simulink model "InnerOuter_Sim"  (Simulink 6.6)
settings: Solver=ode4  StartTime=0.0  StopTime=125  FixedStep=SampleT  RelTol=1e-3
InitFcn:
  | clc
  | innerOuterInit
undefined symbols (not defined in the file): A1, Apolar, apSampleTime, bankCommandLimit, baseHeight, baseTemp, CD0, chord, CL0, CLa, CLa_dot, Clb, ClDa, CLDe, CLDf, ClDr, clock, Clp, CLq, Clr, Cm0, Cma, CmDe, CmDf, Cmq, Cnb, CnDa, CnDr, Cnp, Cnr, compensatorOn, CYb, CYDr, da_failamp, da_failbias, da_failper, daL_fail, daLimit, daR_fail, deg, deLimit, derivativesConstant, dr_fail, dr_failamp, dr_failbias, dr_failper, drLimit, dtLimit, Earth, elarm, Euler_0, F, gaind, getWP, ISA_g, Ixx, Iyy, Izz, L1OF, L2_base ... (+28)
libraries: simulink x102, SLUGS_Library x23, aerolibconvert2 x15, dsPICdrivers x8, aerolibactuator x5, aerolibtransform2 x2, aerolibwind2 x2, dspmtrx3 x2, aerolibatmos2 x1, aerolibutil x1
(part 3 of 4)

== system InnerOuter_Sim/L1 Output Feedback Controller With  Projection Operator/State Predictor/Compute Coef ==
  a : Inport
  Enable : EnablePort
  -T : Gain  Gain=-apSampleTime  SampleTime=apSampleTime
  1-c : Sum  Inputs=-+  OutDataTypeMode=single  OutScaling=2^-10
  Constant : Constant
  Subsystem11 : Subsystem  AncestorBlock=SLUGS_Library/Subsystem11
  b : Outport
  c : Outport  Port=2
  wires:
  -T/1 -> Subsystem11/1(u)
  Subsystem11/1(exp(u)) -> 1-c/1, c/1  "c"
  Constant/1 -> 1-c/2
  1-c/1 -> b/1
  a/1 -> -T/1

== system InnerOuter_Sim/L1 Output Feedback Controller With  Projection Operator/State Predictor/Detect Change ==
  Data : Inport
  Abs1 : Abs  SampleTime=apSampleTime
  Difference1 : simulink/Discrete/Difference  SystemSampleTime=-1  ICPrevInput=0.0  OutDataType=sfix(16)  OutScaling=2^-10  DoSatur=off
  Saturation1 : Saturate  UpperLimit=1  LowerLimit=0  SampleTime=apSampleTime
  change? : Outport
  wires:
  Difference1/1 -> Abs1/1
  Abs1/1 -> Saturation1/1
  Data/1 -> Difference1/1
  Saturation1/1 -> change?/1

== system InnerOuter_Sim/L1 Output Feedback Controller With  Projection Operator/Trapezoidal Integrator/Protect NaNs ==
  In1 : Inport
  Integer Delay3 : simulink/Discrete/Integer Delay  Orientation=left  vinit=0.0  samptime=T  NumDelays=1
  Relational Operator2 : RelationalOperator  Operator===  LogicOutDataTypeMode=Specify via dialog
  Switch3 : Switch  Criteria=u2 > Threshold  Threshold=0.3  SampleTime=.01
  Out1 : Outport  Orientation=down
  wires:
  Integer Delay3/1 -> Switch3/3
  Switch3/1 -> Out1/1, Integer Delay3/1
  In1/1 -> Relational Operator2/2, Relational Operator2/1, Switch3/1
  Relational Operator2/1 -> Switch3/2

== system InnerOuter_Sim/L1 Output Feedback Controller With  Projection Operator/Trapezoidal Integrator/Protect NaNs1 ==
  In1 : Inport
  Integer Delay3 : simulink/Discrete/Integer Delay  Orientation=left  vinit=0.0  samptime=T  NumDelays=1
  Relational Operator2 : RelationalOperator  Operator===  LogicOutDataTypeMode=Specify via dialog
  Switch3 : Switch  Criteria=u2 > Threshold  Threshold=0.3  SampleTime=.01
  Out1 : Outport  Orientation=down
  wires:
  Relational Operator2/1 -> Switch3/2
  In1/1 -> Switch3/1, Relational Operator2/1, Relational Operator2/2
  Switch3/1 -> Integer Delay3/1, Out1/1
  Integer Delay3/1 -> Switch3/3

== system InnerOuter_Sim/Lateral Channel/Sideslip Compensation/Bank to Psi Dot ==
  phi_c : Inport
  U_m : Inport  Port=2
  Constant1 : Constant  Value=9.80665  OutDataTypeMode=single
  Divide : Product  Inputs=/*  OutDataTypeMode=single  OutScaling=2^-10  SampleTime=apSampleTime
  Divide1 : Product  OutDataTypeMode=single  OutScaling=2^-10  SampleTime=apSampleTime
  Subsystem8 : SLUGS_Library/Subsystem8  SystemSampleTime=-1
  negprotect : Stateflow chart
  psi_dot_c : Outport
  wires:
  negprotect/1(zpVal) -> Divide/1
  Divide/1 -> Divide1/2
  phi_c/1 -> Subsystem8/1
  Subsystem8/1 -> Divide1/1
  Divide1/1 -> psi_dot_c/1
  Constant1/1 -> Divide/2
  U_m/1 -> negprotect/1(val)

== system InnerOuter_Sim/Lateral Channel/Sideslip Compensation/Low Pass ==
  a : Inport
  u : Inport  Port=2
  Compute Coef : Subsystem
  Detect Change : Subsystem
  Divide : Product  OutScaling=2^-10  SampleTime=apSampleTime
  Divide1 : Product  OutScaling=2^-10  SampleTime=apSampleTime
  IC : InitialCondition
  Integer Delay : simulink/Discrete/Integer Delay  vinit=0.0  samptime=apSampleTime  NumDelays=1
  Integer Delay1 : simulink/Discrete/Integer Delay  Orientation=left  vinit=0.0  samptime=apSampleTime  NumDelays=1
  Subtract : Sum  OutScaling=2^-10  SampleTime=apSampleTime
  y : Outport
  wires:
  a/1 -> Compute Coef/1(a), Detect Change/1(Data)
  Compute Coef/1(b) -> Divide/1
  Compute Coef/2(c) -> Divide1/1
  Detect Change/1(change?) -> IC/1
  Integer Delay/1 -> Divide/2
  Divide/1 -> Subtract/1
  Divide1/1 -> Subtract/2
  Subtract/1 -> y/1, Integer Delay1/1
  IC/1 -> Compute Coef/Enable
  u/1 -> Integer Delay/1
  Integer Delay1/1 -> Divide1/2

== system InnerOuter_Sim/Lateral Channel/Sideslip Compensation/psi_dot to Bank ==
  psi_dot_c : Inport
  U_m : Inport  Port=2
  Constant1 : Constant  Value=9.80665  OutDataTypeMode=single
  Divide : Product  Inputs=**/  OutScaling=2^-10  SampleTime=apSampleTime
  Subsystem2 : SLUGS_Library/Subsystem2  SystemSampleTime=-1
  phi_c : Outport
  wires:
  Divide/1 -> Subsystem2/1
  Subsystem2/1 -> phi_c/1
  Constant1/1 -> Divide/3
  U_m/1 -> Divide/2
  psi_dot_c/1 -> Divide/1

== system InnerOuter_Sim/Longitudinal Channel/Airspeed Hold [PID]/Trapezoidal Integrator ==
  x : Inport
  Reset : Inport  Port=2
  Constant : Constant  Value=1/3  OutDataTypeMode=single
  Constant1 : Constant  Value=4/3  OutDataTypeMode=single
  Constant2 : Constant  Value=T/2  OutDataTypeMode=single
  Constant3 : Constant  Value=1/3  OutDataTypeMode=single
  Constant5 : Constant  Orientation=left  Value=0  OutDataTypeMode=single
  Integer Delay : simulink/Discrete/Integer Delay  vinit=0.0  samptime=T  NumDelays=1
  Integer Delay1 : simulink/Discrete/Integer Delay  vinit=0.0  samptime=T  NumDelays=2
  Integer Delay2 : simulink/Discrete/Integer Delay  Orientation=left  vinit=0.0  samptime=T  NumDelays=1
  Product{,1..3} (4 alike) : Product  OutDataTypeMode=single  RndMeth=Zero
  "Protect NaNs " : Subsystem
  Protect NaNs1 : Subsystem
  Subtract : Sum  Inputs=3  OutDataTypeMode=single  OutScaling=2^-10
  Subtract1 : Sum  Inputs=2  OutDataTypeMode=single  OutScaling=2^-10
  Switch1 : Switch  Criteria=u2 > Threshold  Threshold=0.3  SampleTime=.01
  Int(x) : Outport
  wires:
  Switch1/1 -> Protect NaNs1/1(In1)
  Reset/1 -> Switch1/2
  Constant5/1 -> Switch1/1
  Product3/1 -> Subtract1/2
  Integer Delay2/1 -> Subtract1/1
  Subtract1/1 -> Switch1/3
  Subtract/1 -> Product3/2
  Constant2/1 -> Product3/1
  Product2/1 -> Subtract/3
  Product1/1 -> Subtract/2
  Product/1 -> Subtract/1
  x/1 -> "Protect NaNs "/1(In1)
  Constant3/1 -> Product2/2
  Integer Delay1/1 -> Product2/1
  Integer Delay/1 -> Product1/1
  Constant1/1 -> Product1/2
  Constant/1 -> Product/2
  Protect NaNs1/1(Out1) -> Integer Delay2/1, Int(x)/1
  "Protect NaNs "/1(Out1) -> Integer Delay1/1, Integer Delay/1, Product/1

== system InnerOuter_Sim/Navigation/Compute WP Switching Trigger/Compute  Projection ==
  Puav : Inport
  WP0 : Inport  Port=2
  T : Inport  Port=3
  Protect NaNs : Subsystem
  Subsystem3 : Subsystem  AncestorBlock=SLUGS_Library/Subsystem3
  Subtract : Sum  Inputs=+-  OutDataTypeMode=single  OutScaling=2^-10
  Dg : Outport
  wires:
  Protect NaNs/1(Out1) -> Dg/1
  Puav/1 -> Subtract/1
  WP0/1 -> Subtract/2
  Subtract/1 -> Subsystem3/1(x)
  T/1 -> Subsystem3/2(y)
  Subsystem3/1(x dot y) -> Protect NaNs/1(In1)

== system InnerOuter_Sim/Navigation/Leg Run Computation/Compute Lateral Error ==
  N1 : Inport
  WP0 : Inport  Port=2
  Puav : Inport  Port=3
  Add : Sum  Inputs=+-  OutScaling=2^-10
  Subsystem3 : SLUGS_Library/Subsystem3  SystemSampleTime=-1
  Pe_y : Outport
  wires:
  Subsystem3/1 -> Pe_y/1
  Add/1 -> Subsystem3/2
  N1/1 -> Subsystem3/1
  Puav/1 -> Add/2
  WP0/1 -> Add/1

== system InnerOuter_Sim/Navigation/Leg Run Computation/GainSchedule L2 and Get Groundspeed ==
  L2 Base : Inport
  Vxyz : Inport  Port=2
  Divide4 : Product  OutScaling=2^-10
  "Norm 2 (Consider Only XY) " : Subsystem  AncestorBlock=SLUGS_Library/Navigation/Norm
  To Workspace3 : ToWorkspace  VariableName=L2  SampleTime=-1  SaveFormat=Array
  L2 : Outport
  Groundspeed : Outport  Port=2
  wires:
  "Norm 2 (Consider Only XY) "/1(Norm) -> Groundspeed/1, Divide4/2
  Vxyz/1 -> "Norm 2 (Consider Only XY) "/1(Vector)
  L2 Base/1 -> Divide4/1
  Divide4/1 -> L2/1, To Workspace3/1

== system InnerOuter_Sim/Navigation/Leg Run Computation/Pey <= |L2| (Park and Deyst's) ==
  Pey : Inport
  Vxyz : Inport  Port=2
  L2 : Inport  Port=3
  T1 : Inport  Port=4
  Groundspeed : Inport  Port=5
  Puav : Inport  Port=6
  N1 : Inport  Port=7
  Enable : EnablePort
  Add : Sum  Inputs=+-  OutScaling=2^-10
  Compute D : Subsystem
  Compute Eta : Subsystem
  Gravity1 : Constant  Orientation=left  Value=ISA_g  OutDataTypeMode=single
  Zero out Z : Stateflow chart
  as_c to phi_c1 : Subsystem  AncestorBlock=SLUGS_Library/Navigation/as_c to phi_c
  phi_c : Outport
  L2Vec : Outport  Port=2
  as_c : Outport  Port=3
  wires:
  Compute D/1(D) -> Add/1
  Zero out Z/1(P) -> Add/2, Compute D/4(Puav)
  Vxyz/1 -> Compute Eta/1(Vxyz)
  Add/1 -> Compute Eta/2(L2vec), L2Vec/1
  Gravity1/1 -> as_c to phi_c1/2(g)
  Compute Eta/1(a_s_c) -> as_c to phi_c1/1(as_c), as_c/1
  Pey/1 -> Compute D/1(Pe_y)
  L2/1 -> Compute D/2(|L2|), Compute Eta/4(|L2|)
  Puav/1 -> Zero out Z/1(Pin)
  T1/1 -> Compute D/3(T1)
  Groundspeed/1 -> Compute Eta/3(Groundspeed)
  as_c to phi_c1/1(phi_c) -> phi_c/1
  N1/1 -> Compute D/5(N1)

== system InnerOuter_Sim/Navigation/Leg Run Computation/Pey > |L2| (Marius') ==
  Pey : Inport
  Kr : Inport  Port=2
  T1 : Inport  Port=3
  Tot Run : Inport  Port=4
  Puav : Inport  Port=5
  WP0 : Inport  Port=6
  U_m : Inport  Port=7
  Enable : EnablePort
  Add1 : Sum  Inputs=+-  OutScaling=2^-10
  Add2 : Sum  Inputs=-+  OutScaling=2^-10
  Add3 : Sum  Inputs=-+  OutScaling=2^-10
  Constant1 : Constant  Value=0.0025  OutDataTypeMode=single
  Low_passed Time  Derivative : Subsystem  AncestorBlock="SLUGS_Library/Control Blocks/PD Controller  Internal Derivative/Low_passed Time Derivative"
  Low_passed Time  Derivative1 : Subsystem  AncestorBlock="SLUGS_Library/Control Blocks/PD Controller  Internal Derivative/Low_passed Time Derivative"
  Product : Product  Inputs=3  RndMeth=Zero
  Product1 : Product  RndMeth=Zero
  Product2 : Product  RndMeth=Zero
  Subsystem3 : SLUGS_Library/Subsystem3  SystemSampleTime=-1
  Zero out Z : Stateflow chart
  Zero out Z1 : Stateflow chart
  psi_dot to Bank : Subsystem  AncestorBlock=SLUGS_Library/Navigation/psi_dot to Bank
  phi_c : Outport
  wires:
  Puav/1 -> Add1/1
  WP0/1 -> Add1/2
  Add1/1 -> Zero out Z1/1(Pin)
  T1/1 -> Zero out Z/1(Pin)
  Tot Run/1 -> Add2/2
  psi_dot to Bank/1(phi_c) -> phi_c/1
  Add2/1 -> Product/1, Low_passed Time  Derivative/1(f(t))  "xTrack"
  Pey/1 -> Product1/2, Low_passed Time  Derivative1/1(f(t))  "yTreack"
  Low_passed Time  Derivative1/1(f_dot(t)) -> Product/2
  Kr/1 -> Product/3
  Low_passed Time  Derivative/1(f_dot(t)) -> Product1/1
  Product1/1 -> Add3/1
  Product/1 -> Add3/2
  U_m/1 -> psi_dot to Bank/2(U_m)
  Subsystem3/1 -> Add2/1
  Zero out Z/1(P) -> Subsystem3/1  "Pex"
  Zero out Z1/1(P) -> Subsystem3/2
  Product2/1 -> psi_dot to Bank/1(psi_dot_c)
  Add3/1 -> Product2/2
  Constant1/1 -> Product2/1

== system InnerOuter_Sim/Navigation/Leg Run Computation/Record Data ==
  ApMode : Inport
  "L2Vec " : Inport  Port=2
  as_c : Inport  Port=3
  "ApMode " : InportShadow  Port=1  LatchByCopyingInsideSignal=off
  Constant2 : Constant  Value=[0 0 0]  OutDataTypeMode=single
  Switch : Switch  Threshold=0.3
  Switch1 : Switch  Threshold=0.3
  L2Vec : Outport
  "as_c " : Outport  Port=2
  wires:
  Switch/1 -> L2Vec/1
  Constant2/1 -> Switch/3, Switch1/3
  Switch1/1 -> "as_c "/1
  ApMode/1 -> Switch/2
  "L2Vec "/1 -> Switch/1
  as_c/1 -> Switch1/1
  "ApMode "/1 -> Switch1/2

== system InnerOuter_Sim/Navigation/Mode Determination/Recent Enable ==
  WP Fly : Inport
  Puav : Inport  Port=2
  Data Type Conversion1 : DataTypeConversion  OutDataTypeMode=double  SampleTime=apSampleTime
  Grab Upon Enable : Subsystem  TreatAsAtomicUnit=on
  IC1 : InitialCondition  Value=0
  Subsystem : Subsystem
  UAV IC : Outport
  WPEnable : Outport  Port=2
  wires:
  IC1/1 -> Subsystem/1(WP Fly)
  Grab Upon Enable/1(UAVic) -> UAV IC/1
  Puav/1 -> Grab Upon Enable/1(Puav)
  Subsystem/1(Just Enab) -> Grab Upon Enable/Enable, WPEnable/1
  WP Fly/1 -> Data Type Conversion1/1
  Data Type Conversion1/1 -> IC1/1

== system InnerOuter_Sim/Navigation/Waypoint Transition Computation/Compute P ==
  T1 : Inport
  T2 : Inport  Port=2
  WP1 : Inport  Port=3
  U_comm : Inport  Port=4
  Preturn K : Inport  Port=5
  Groundspeed : Inport  Port=6
  Add : Sum  Inputs=2  OutScaling=2^-10
  Compute R : Subsystem
  Get Circles : Subsystem
  Product1 : Product  OutDataTypeMode=single  RndMeth=Zero
  To Workspace : ToWorkspace  VariableName=R1  SampleTime=-1  SaveFormat=Structure
  P : Outport
  wires:
  WP1/1 -> Get Circles/3("Wp_to ")
  T1/1 -> Get Circles/1(T1)
  Add/1 -> P/1
  Get Circles/1(P) -> Add/2
  Product1/1 -> Add/1
  T2/1 -> Get Circles/2(T2)
  Preturn K/1 -> Product1/1
  Groundspeed/1 -> Product1/2
  Compute R/1(R) -> Get Circles/4(R), To Workspace/1
  U_comm/1 -> Compute R/1(U_com)

== system InnerOuter_Sim/Navigation/Waypoint Transition Computation/Compute Total Run ==
  P : Inport
  "WP0  " : Inport  Port=2
  WP1 : Inport  Port=3
  Compute Distance : Subsystem
  Protect NaNs : Subsystem
  Subtract1 : Sum  Inputs=-+  OutDataTypeMode=single  OutScaling=2^-10
  Tot Run : Outport  InitialOutput=150
  wires:
  Protect NaNs/1(Out1) -> Tot Run/1
  WP1/1 -> Compute Distance/2(Pos 2)
  "WP0  "/1 -> Compute Distance/1(Pos 1)
  Compute Distance/1(Dist) -> Subtract1/2
  P/1 -> Subtract1/1
  Subtract1/1 -> Protect NaNs/1(In1)

== system InnerOuter_Sim/Navigation/Waypoint Transition Computation/Get Wps Compute Frenet1 ==
  WP Idx 0 : Inport
  WP Idx 1 : Inport  Port=2
  WP Idx 2 : Inport  Port=3
  UAV IC : Inport  Port=4
  Compute Frenet : Subsystem  AncestorBlock=SLUGS_Library/Navigation/Compute Frenet
  "Compute Frenet " : Subsystem  AncestorBlock=SLUGS_Library/Navigation/Compute Frenet
  Display : Display
  Display1 : Display
  Display2 : Display
  Switch : Switch  Criteria=u2 > Threshold  Threshold=0.3  ZeroCross=off
  Terminator : Terminator
  get WP Coord from Index : Subsystem  AncestorBlock=SLUGS_Library/Navigation/get WP Coord from Index
  "get WP Coord from Index " : Subsystem  AncestorBlock=SLUGS_Library/Navigation/get WP Coord from Index
  "get WP Coord from Index   " : Subsystem  AncestorBlock=SLUGS_Library/Navigation/get WP Coord from Index
  T1 : Outport
  N1 : Outport  Port=2
  T2 : Outport  Port=3
  WP0 : Outport  Port=4
  WP 1 : Outport  Orientation=left  Port=5
  wires:
  "Compute Frenet "/2(N) -> Terminator/1
  "Compute Frenet "/1(T) -> T2/1
  "get WP Coord from Index   "/1(WP Coord) -> "Compute Frenet "/2(Pos 2)
  WP Idx 2/1 -> "get WP Coord from Index   "/1(WP Idx)
  UAV IC/1 -> Switch/3, Display1/1
  get WP Coord from Index/1(WP Coord) -> Switch/1
  Switch/1 -> Compute Frenet/1(Pos 1), WP0/1, Display/1
  "get WP Coord from Index "/1(WP Coord) -> WP 1/1, "Compute Frenet "/1(Pos 1), Compute Frenet/2(Pos 2)
  WP Idx 1/1 -> "get WP Coord from Index "/1(WP Idx)
  Compute Frenet/2(N) -> N1/1
  Compute Frenet/1(T) -> T1/1
  WP Idx 0/1 -> get WP Coord from Index/1(WP Idx), Switch/2, Display2/1

== system InnerOuter_Sim/6DOF Model/Plant/6-DOF EOM/Get Euler Dot ==
  p,q,r : Inport
  Euler : Inport  Port=2
  Mux1 : Mux  Inputs=[3 3]
  Mux2 : Mux  Inputs=3
  phidot : Fcn  Expr=u[1]+u[2]*sin(u[4])*tan(u[5])+u[3]*cos(u[4])*tan(u[5])
  psidot : Fcn  Expr=u[2]*sin(u[4])/cos(u[5])+u[3]*cos(u[4])/cos(u[5])
  thetadot : Fcn  Expr=u[2]*cos(u[4])-u[3]*sin(u[4])
  Euler_dot : Outport
  wires:
  Mux2/1 -> Euler_dot/1
  phidot/1 -> Mux2/1
  thetadot/1 -> Mux2/2
  psidot/1 -> Mux2/3
  Mux1/1 -> thetadot/1, phidot/1, psidot/1
  p,q,r/1 -> Mux1/1
  Euler/1 -> Mux1/2

== system InnerOuter_Sim/6DOF Model/Plant/6-DOF EOM/RB2LTP ==
  Euler : Inport
  11 : Fcn  Expr=cos(u[3])*cos(u[2])
  12 : Fcn  Expr=sin(u[3])*cos(u[2])
  13 : Fcn  Expr=-sin(u[2])
  21 : Fcn  Expr=cos(u[3])*sin(u[2])*sin(u[1])-sin(u[3])*cos(u[1])
  22 : Fcn  Expr=sin(u[3])*sin(u[2])*sin(u[1])+cos(u[3])*cos(u[1])
  23 : Fcn  Expr=cos(u[2])*sin(u[1])
  31 : Fcn  Expr=cos(u[3])*sin(u[2])*cos(u[1])+sin(u[3])*sin(u[1])
  32 : Fcn  Expr=sin(u[3])*sin(u[2])*cos(u[1])-cos(u[3])*sin(u[1])
  33 : Fcn  Expr=cos(u[2])*cos(u[1])
  Mux2 : Mux  Inputs=9
  Reshape : Reshape  OutputDimensionality=Customize  OutputDimensions=[3,3]
  Rot : Outport
  wires:
  33/1 -> Mux2/9
  32/1 -> Mux2/8
  31/1 -> Mux2/7
  23/1 -> Mux2/6
  22/1 -> Mux2/5
  21/1 -> Mux2/4
  13/1 -> Mux2/3
  12/1 -> Mux2/2
  11/1 -> Mux2/1
  Mux2/1 -> Reshape/1
  Euler/1 -> 11/1, 33/1, 32/1, 31/1, 23/1, 22/1, 21/1, 13/1, 12/1
  Reshape/1 -> Rot/1

== system InnerOuter_Sim/6DOF Model/Plant/6-DOF EOM/[V1,2,3,W1,2,3] ==
  note: V*dot =Inv(A){[F ; M] - SigmaAV*}
  "[F ; M]" : Inport
  Euler : Inport  Port=2
  V* : Inport  Port=3  PortDimensions=6
  A = [M ; J] : Subsystem
  Acc_meas : Product  Inputs=/*  Multiplication=Matrix(*)  SaturateOnIntegerOverflow=on  InputSameDT=on
  Demux : Demux  Outputs=[3;3]
  Get Grav Force in Body : Subsystem
  Gravitational Acc : Constant  Value=[0 0 -ISA_g]  VectorParams1D=off
  Selector3 : Selector  IndexOptions=Index vector (dialog)  Indices=1:3  OutputSizes=1  InputPortWidth=6
  Sigma : Subsystem
  Sigma*A : Product  Multiplication=Matrix(*)  SaturateOnIntegerOverflow=on  InputSameDT=on
  Sigma*A*V* : Product  Multiplication=Matrix(*)  SaturateOnIntegerOverflow=on  InputSameDT=on
  Sum1 : Sum  Inputs=+-|  SaturateOnIntegerOverflow=on  InputSameDT=on
  Sum2 : Sum  Inputs=++|  SaturateOnIntegerOverflow=on  InputSameDT=on
  Terminator1 : Terminator
  "V*dot " : Product  Inputs=/*  Multiplication=Matrix(*)  SaturateOnIntegerOverflow=on  InputSameDT=on
  "Acc_meas " : Outport
  V*dot : Outport  Port=2
  wires:
  Sum2/1 -> "Acc_meas "/1
  Get Grav Force in Body/1(Grav Force (Body)) -> Sum2/1
  Selector3/1 -> Sum2/2
  Euler/1 -> Get Grav Force in Body/1(Euler)
  Gravitational Acc/1 -> Get Grav Force in Body/2(Grav Force)
  Acc_meas/1 -> Selector3/1
  Sigma*A/1 -> Sigma*A*V*/1
  "V*dot "/1 -> V*dot/1
  V*/1 -> Demux/1, Sigma*A*V*/2
  Demux/2 -> Sigma/1(pqr)
  Sigma*A*V*/1 -> Sum1/2
  "[F ; M]"/1 -> Acc_meas/2, Sum1/1
  Sigma/1(Sigma) -> Sigma*A/1
  Demux/1 -> Terminator1/1
  A = [M ; J]/1(A Matrix) -> Acc_meas/1, "V*dot "/1, Sigma*A/2
  Sum1/1 -> "V*dot "/2

== system InnerOuter_Sim/6DOF Model/Plant/Engine Model/Get To1 ==
  dt : Inport
  Divide : Product  Inputs=3  OutScaling=2^-10
  Math Function : Math  Operator=pow  SaturateOnIntegerOverflow=on
  Math Function1 : Math  Operator=pow  SaturateOnIntegerOverflow=on
  MaxRPM : Gain  Gain=7200  SaturateOnIntegerOverflow=on
  Min RPM : Constant  Value=2000
  Min Th K : Constant  Value=MinThK
  Prop Diameter (in) : Constant  Value=17
  Prop Diameter (in)1 : Constant  Value=2
  Prop Diameter (in)2 : Constant  Value=4
  Saturation : Saturate  UpperLimit=1.0  LowerLimit=0
  Sum : Sum  Inputs=|++
  Sum1 : Sum  Inputs=|++
  TFact : simulink/Math Operations/Slider Gain  SystemSampleTime=-1  low=0  gain=0.2  high=1
  Th K : Gain  Gain=ThK  SaturateOnIntegerOverflow=on
  To Constant : Constant  Value=2.83e-12
  To : Outport
  wires:
  Saturation/1 -> Th K/1
  Prop Diameter (in)1/1 -> Math Function/2
  Prop Diameter (in)2/1 -> Math Function1/2
  Prop Diameter (in)/1 -> Math Function1/1
  Math Function/1 -> Divide/1
  Math Function1/1 -> Divide/2
  To Constant/1 -> Divide/3
  Divide/1 -> TFact/1
  TFact/1 -> To/1
  Sum/1 -> Math Function/1
  Min RPM/1 -> Sum/2
  MaxRPM/1 -> Sum/1
  Th K/1 -> Sum1/1
  dt/1 -> Saturation/1
  Sum1/1 -> MaxRPM/1
  Min Th K/1 -> Sum1/2

== system InnerOuter_Sim/6DOF Model/Plant/Forces and Moments/Alpha/Beta ==
  "Vx, Vy, Vz (Body)" : Inport
  Rho : Inport  Port=2
  Constant : Constant  Value=0.5  VectorParams1D=off
  Math Function : Math  Operator=sqrt  SaturateOnIntegerOverflow=on
  Product : Product  Inputs=3  SaturateOnIntegerOverflow=on
  Product1 : Product  Inputs=3  SaturateOnIntegerOverflow=on
  R2D1 : Gain  Gain=180/pi  SaturateOnIntegerOverflow=on
  R2D2 : Gain  Gain=180/pi  SaturateOnIntegerOverflow=on
  V^2 : Fcn  Expr=(u(1)^2+u(2)^2+u(3)^2)
  "[-15; 15 ]" : Saturate  UpperLimit=15  LowerLimit=-15
  "[-15;15]" : Saturate  UpperLimit=15  LowerLimit=-15
  aoa : Trigonometry  Operator=asin
  beta : Trigonometry  Operator=atan
  sin(aoa) : Fcn  Expr=u(3)/sqrt(u(1)^2+u(3)^2)
  span : Constant  Value=span  VectorParams1D=off
  span1 : Constant  Value=chord  VectorParams1D=off
  tan(beta) : Fcn  Expr=u(2)/sqrt(u(1)^2+u(3)^2)
  "alpha, deg" : Outport
  "beta, deg" : Outport  Port=2
  qS : Outport  Port=3
  Speed : Outport  Port=4
  q : Outport  Port=5
  wires:
  Product/1 -> q/1, Product1/1
  Product1/1 -> qS/1
  span1/1 -> Product1/3
  span/1 -> Product1/2
  "Vx, Vy, Vz (Body)"/1 -> sin(aoa)/1, V^2/1, tan(beta)/1
  tan(beta)/1 -> beta/1
  beta/1 -> R2D1/1
  V^2/1 -> Product/1, Math Function/1
  Rho/1 -> Product/2
  Constant/1 -> Product/3
  R2D1/1 -> "[-15; 15 ]"/1  "beta"
  aoa/1 -> R2D2/1
  R2D2/1 -> "[-15;15]"/1  "aoa"
  sin(aoa)/1 -> aoa/1
  Math Function/1 -> Speed/1
  "[-15;15]"/1 -> "alpha, deg"/1
  "[-15; 15 ]"/1 -> "beta, deg"/1

== system InnerOuter_Sim/6DOF Model/Plant/Forces and Moments/Body Frame F & M ==
  "Alpha, deg" : Inport
  "Beta, deg" : Inport  Port=2
  qs : Inport  Port=3
  Airspeed : Inport  Port=4
  "de, deg" : Inport  Port=5
  "daL, deg" : Inport  Port=6
  "daR, deg" : Inport  Port=7
  "dr, deg" : Inport  Port=8
  "df, deg" : Inport  Port=9
  p,q,r : Inport  Port=10
  Bus Creator : BusCreator  Inputs=2
  Transfer to body frame : Subsystem
  Wind frame F& M : Subsystem
  F_b : Outport
  M_b : Outport  Port=2
  wires:
  "Alpha, deg"/1 -> Wind frame F& M/1("alpha, deg"), Bus Creator/1
  "Beta, deg"/1 -> Wind frame F& M/2("beta, deg"), Bus Creator/2
  "dr, deg"/1 -> Wind frame F& M/6("dr, deg")
  "daL, deg"/1 -> Wind frame F& M/4("daL, deg")
  "de, deg"/1 -> Wind frame F& M/3("de, deg")
  Wind frame F& M/1(F&M wind frame) -> Transfer to body frame/1(Wind frame  F&M)
  Bus Creator/1 -> Transfer to body frame/2("aoa/beta, deg")  "aoa/beta, deg"
  Transfer to body frame/1(F_b) -> F_b/1
  Transfer to body frame/2(M_b) -> M_b/1
  "df, deg"/1 -> Wind frame F& M/7("df, deg")
  qs/1 -> Wind frame F& M/8(qS)
  p,q,r/1 -> Wind frame F& M/9(p,q,r)
  Airspeed/1 -> Wind frame F& M/10(Airpseed)
  "daR, deg"/1 -> Wind frame F& M/5("daR, deg")

== system InnerOuter_Sim/6DOF Model/Plant/Forces and Moments/Get Grav Force in Body ==
  Euler : Inport
  Grav Force : Inport  Port=2
  Math Function : Math  Operator=transpose  SaturateOnIntegerOverflow=on
  Product1 : Product  Multiplication=Matrix(*)  SaturateOnIntegerOverflow=on  InputSameDT=on
  Rb2u : Subsystem
  Reshape : Reshape  OutputDimensionality=Column vector (2-D)
  Grav Force (Body) : Outport
  wires:
  Rb2u/1(DCM) -> Math Function/1
  Euler/1 -> Rb2u/1(phi theta psi)
  Product1/1 -> Grav Force (Body)/1
  Math Function/1 -> Product1/1
  Grav Force/1 -> Reshape/1
  Reshape/1 -> Product1/2

== system InnerOuter_Sim/6DOF Model/Plant/Forces and Moments/NED(u)2b ==
  V w : Inport
  Euler : Inport  Port=2
  RB2LTP : Subsystem
  RL2B * Vw : Product  Multiplication=Matrix(*)  SaturateOnIntegerOverflow=on  InputSameDT=on
  RLTP2B : Math  Operator=transpose  SaturateOnIntegerOverflow=on
  Reshape1 : Reshape  OutputDimensionality=Row vector (2-D)
  Vb Corr : Outport
  wires:
  RL2B * Vw/1 -> Reshape1/1
  Euler/1 -> RB2LTP/1(Euler)
  RB2LTP/1(RB2L) -> RLTP2B/1
  RLTP2B/1 -> RL2B * Vw/1
  V w/1 -> RL2B * Vw/2
  Reshape1/1 -> Vb Corr/1

== system InnerOuter_Sim/6DOF Model/Plant/Magnetometer/RB2LTP ==
  Euler : Inport
  11 : Fcn  Expr=cos(u[3])*cos(u[2])
  12 : Fcn  Expr=sin(u[3])*cos(u[2])
  13 : Fcn  Expr=-sin(u[2])
  21 : Fcn  Expr=cos(u[3])*sin(u[2])*sin(u[1])-sin(u[3])*cos(u[1])
  22 : Fcn  Expr=sin(u[3])*sin(u[2])*sin(u[1])+cos(u[3])*cos(u[1])
  23 : Fcn  Expr=cos(u[2])*sin(u[1])
  31 : Fcn  Expr=cos(u[3])*sin(u[2])*cos(u[1])+sin(u[3])*sin(u[1])
  32 : Fcn  Expr=sin(u[3])*sin(u[2])*cos(u[1])-cos(u[3])*sin(u[1])
  33 : Fcn  Expr=cos(u[2])*cos(u[1])
  Mux2 : Mux  Inputs=9
  Reshape : Reshape  OutputDimensionality=Customize  OutputDimensions=[3,3]
  Rot : Outport
  wires:
  33/1 -> Mux2/9
  32/1 -> Mux2/8
  31/1 -> Mux2/7
  23/1 -> Mux2/6
  22/1 -> Mux2/5
  21/1 -> Mux2/4
  13/1 -> Mux2/3
  12/1 -> Mux2/2
  11/1 -> Mux2/1
  Mux2/1 -> Reshape/1
  Euler/1 -> 11/1, 33/1, 32/1, 31/1, 23/1, 22/1, 21/1, 13/1, 12/1
  Reshape/1 -> Rot/1

== system InnerOuter_Sim/6DOF Model/Plant/[0, pi] Wrap Around/Negative Yaw ==
  yaw : Inport
  Enable : EnablePort
  Abs : Abs
  Constant1 : Constant  Value=2*pi
  Constant2 : Constant  Value=2*pi
  Math Function : Math  Operator=mod  SaturateOnIntegerOverflow=on
  Sum : Sum  Inputs=|-+
  yaw_wr : Outport
  wires:
  yaw/1 -> Abs/1
  Constant1/1 -> Math Function/2
  Math Function/1 -> Sum/1
  Abs/1 -> Math Function/1
  Constant2/1 -> Sum/2
  Sum/1 -> yaw_wr/1

== system InnerOuter_Sim/6DOF Model/Plant/[0, pi] Wrap Around/Positive Yaw ==
  yaw : Inport
  Enable : EnablePort
  Constant1 : Constant  Value=2*pi
  Math Function : Math  Operator=mod  SaturateOnIntegerOverflow=on
  yaw_wr : Outport
  wires:
  yaw/1 -> Math Function/1
  Constant1/1 -> Math Function/2
  Math Function/1 -> yaw_wr/1

== system InnerOuter_Sim/L1 Output Feedback Controller With  Projection Operator/Control  Law/Compute Coef/Subsystem11 ==
  u : Inport
  Environment Controller : simulink/Signal Routing/Environment Controller  SystemSampleTime=-1
  Math Function : Math  SaturateOnIntegerOverflow=on
  exp(u) : Outport
  wires:
  Environment Controller/1 -> exp(u)/1
  Math Function/1 -> Environment Controller/1
  u/1 -> Math Function/1

== system InnerOuter_Sim/L1 Output Feedback Controller With  Projection Operator/State Predictor/Compute Coef/Subsystem11 ==
  u : Inport
  Environment Controller : simulink/Signal Routing/Environment Controller  SystemSampleTime=-1
  Math Function : Math  SaturateOnIntegerOverflow=on
  exp(u) : Outport
  wires:
  Environment Controller/1 -> exp(u)/1
  Math Function/1 -> Environment Controller/1
  u/1 -> Math Function/1

== system InnerOuter_Sim/Lateral Channel/Sideslip Compensation/Low Pass/Compute Coef ==
  a : Inport
  Enable : EnablePort
  -T : Gain  Gain=-apSampleTime  SampleTime=apSampleTime
  1-c : Sum  Inputs=-+  OutDataTypeMode=single  OutScaling=2^-10  SampleTime=apSampleTime
  Constant : Constant
  Math Function : Math  SaturateOnIntegerOverflow=on
  b : Outport
  c : Outport  Port=2
  wires:
  -T/1 -> Math Function/1
  Math Function/1 -> 1-c/1, c/1  "c"
  Constant/1 -> 1-c/2
  1-c/1 -> b/1
  a/1 -> -T/1

== system InnerOuter_Sim/Lateral Channel/Sideslip Compensation/Low Pass/Detect Change ==
  Data : Inport
  Abs1 : Abs  SampleTime=apSampleTime
  Difference1 : simulink/Discrete/Difference  SystemSampleTime=-1  ICPrevInput=0.0  OutDataType=sfix(16)  OutScaling=2^-10  DoSatur=off
  Saturation1 : Saturate  UpperLimit=1  LowerLimit=0  SampleTime=apSampleTime
  change? : Outport
  wires:
  Difference1/1 -> Abs1/1
  Abs1/1 -> Saturation1/1
  Data/1 -> Difference1/1
  Saturation1/1 -> change?/1

== system InnerOuter_Sim/Longitudinal Channel/Airspeed Hold [PID]/Trapezoidal Integrator/Protect NaNs  ==
  In1 : Inport
  Integer Delay3 : simulink/Discrete/Integer Delay  Orientation=left  vinit=0.0  samptime=T  NumDelays=1
  Relational Operator2 : RelationalOperator  Operator===  LogicOutDataTypeMode=Specify via dialog
  Switch3 : Switch  Criteria=u2 > Threshold  Threshold=0.3  SampleTime=.01
  Out1 : Outport  Orientation=down
  wires:
  Integer Delay3/1 -> Switch3/3
  Switch3/1 -> Out1/1, Integer Delay3/1
  In1/1 -> Relational Operator2/2, Relational Operator2/1, Switch3/1
  Relational Operator2/1 -> Switch3/2

== system InnerOuter_Sim/Longitudinal Channel/Airspeed Hold [PID]/Trapezoidal Integrator/Protect NaNs1 ==
  In1 : Inport
  Integer Delay3 : simulink/Discrete/Integer Delay  Orientation=left  vinit=0.0  samptime=T  NumDelays=1
  Relational Operator2 : RelationalOperator  Operator===  LogicOutDataTypeMode=Specify via dialog
  Switch3 : Switch  Criteria=u2 > Threshold  Threshold=0.3  SampleTime=.01
  Out1 : Outport  Orientation=down
  wires:
  Integer Delay3/1 -> Switch3/3
  Switch3/1 -> Out1/1, Integer Delay3/1
  In1/1 -> Relational Operator2/2, Relational Operator2/1, Switch3/1
  Relational Operator2/1 -> Switch3/2

== system InnerOuter_Sim/Navigation/Compute WP Switching Trigger/Compute  Projection/Protect NaNs ==
  In1 : Inport
  Integer Delay3 : simulink/Discrete/Integer Delay  Orientation=left  vinit=0.0  samptime=T  NumDelays=1
  Relational Operator2 : RelationalOperator  Operator===  LogicOutDataTypeMode=Specify via dialog
  Switch3 : Switch  Criteria=u2 > Threshold  Threshold=0.3  SampleTime=.01
  Out1 : Outport  Orientation=down
  wires:
  Integer Delay3/1 -> Switch3/3
  Switch3/1 -> Out1/1, Integer Delay3/1
  In1/1 -> Relational Operator2/2, Relational Operator2/1, Switch3/1
  Relational Operator2/1 -> Switch3/2

== system InnerOuter_Sim/Navigation/Compute WP Switching Trigger/Compute  Projection/Subsystem3 ==
  x : Inport
  y : Inport  Port=2
  Embedded MATLAB Function : Stateflow chart
  x dot y : Outport
  wires:
  y/1 -> Embedded MATLAB Function/2(y)
  x/1 -> Embedded MATLAB Function/1(x)
  Embedded MATLAB Function/1(xDoty) -> x dot y/1

== system InnerOuter_Sim/Navigation/Leg Run Computation/GainSchedule L2 and Get Groundspeed/Norm 2 (Consider Only XY)  ==
  Vector : Inport
  Subsystem1 : Subsystem  AncestorBlock=SLUGS_Library/Subsystem1
  Subsystem3 : Subsystem  AncestorBlock=SLUGS_Library/Subsystem3
  Norm : Outport
  wires:
  Subsystem1/1(sqrt(x)) -> Norm/1
  Vector/1 -> Subsystem3/1(x), Subsystem3/2(y)
  Subsystem3/1(x dot2 y) -> Subsystem1/1(x)

== system InnerOuter_Sim/Navigation/Leg Run Computation/Pey <= |L2| (Park and Deyst's)/Compute D ==
  Pe_y : Inport
  |L2| : Inport  Port=2
  T1 : Inport  Port=3
  Puav : Inport  Port=4
  N1 : Inport  Port=5
  Add1 : Sum  Inputs=2  OutScaling=2^-10
  Add2 : Sum  Inputs=2  OutScaling=2^-10
  Divide : Product  Inputs=*/  OutScaling=2^-10
  Divide1 : Product  Inputs=3  OutScaling=2^-10
  Divide2 : Product  OutScaling=2^-10
  "Pe_y " : InportShadow  Port=1  LatchByCopyingInsideSignal=off
  Subsystem10 : Subsystem  AncestorBlock=SLUGS_Library/Subsystem10
  Subsystem7 : Subsystem  AncestorBlock=SLUGS_Library/Subsystem7
  D : Outport
  wires:
  Divide/1 -> Subsystem10/1(x)
  Subsystem10/1(acos(x)) -> Subsystem7/1(x)  "lambda"
  Subsystem7/1(sin(x)) -> Divide1/1
  |L2|/1 -> Divide/2, Divide1/2
  Pe_y/1 -> Divide/1
  T1/1 -> Divide1/3
  Divide1/1 -> Add1/1  "T . ||CD||"
  "Pe_y "/1 -> Divide2/1
  N1/1 -> Divide2/2
  Divide2/1 -> Add2/1
  Puav/1 -> Add2/2
  Add2/1 -> Add1/2  "Puav + PeyN"
  Add1/1 -> D/1

== system InnerOuter_Sim/Navigation/Leg Run Computation/Pey <= |L2| (Park and Deyst's)/Compute Eta ==
  Vxyz : Inport
  L2vec : Inport  Port=2
  Groundspeed : Inport  Port=3
  |L2| : Inport  Port=4
  3x3 Cross Product : aerolibutil/3x3 Cross Product  SystemSampleTime=-1
  Constant : Constant  Value=2
  Divide5 : Product  Inputs=*//  OutScaling=2^-10
  "Groundspeed " : InportShadow  Port=3  LatchByCopyingInsideSignal=off
  Product : Product  Inputs=***/*  RndMeth=Zero
  Selector : Selector  IndexOptions=Index vector (dialog)  Indices=[3]  OutputSizes=1  InputPortWidth=3
  |L2|1 : InportShadow  Port=4  LatchByCopyingInsideSignal=off
  a_s_c : Outport
  wires:
  Groundspeed/1 -> Divide5/3
  L2vec/1 -> 3x3 Cross Product/2
  Divide5/1 -> Selector/1
  3x3 Cross Product/1 -> Divide5/1
  Vxyz/1 -> 3x3 Cross Product/1
  Selector/1 -> Product/5
  |L2|/1 -> Divide5/2
  Product/1 -> a_s_c/1
  |L2|1/1 -> Product/4
  Constant/1 -> Product/3
  "Groundspeed "/1 -> Product/2, Product/1

== system InnerOuter_Sim/Navigation/Leg Run Computation/Pey <= |L2| (Park and Deyst's)/as_c to phi_c1 ==
  as_c : Inport
  g : Inport  Port=2
  Divide : Product  Inputs=*/  OutScaling=2^-10
  Subsystem2 : SLUGS_Library/Subsystem2  SystemSampleTime=-1
  phi_c : Outport
  wires:
  Divide/1 -> Subsystem2/1
  as_c/1 -> Divide/1
  Subsystem2/1 -> phi_c/1
  g/1 -> Divide/2

== system InnerOuter_Sim/Navigation/Leg Run Computation/Pey > |L2| (Marius')/Low_passed Time  Derivative ==
  f(t) : Inport
  Add : Sum  Inputs=+-  OutScaling=2^-10
  Constant : Constant  Value=5*T  OutDataTypeMode=single
  Divide : Product  Inputs=*/  OutScaling=2^-10
  Integer Delay : simulink/Discrete/Integer Delay  vinit=0.0  samptime=T  NumDelays=5
  f_dot(t) : Outport
  wires:
  Divide/1 -> f_dot(t)/1
  Constant/1 -> Divide/2
  Integer Delay/1 -> Add/2
  f(t)/1 -> Integer Delay/1, Add/1
  Add/1 -> Divide/1

== system InnerOuter_Sim/Navigation/Leg Run Computation/Pey > |L2| (Marius')/Low_passed Time  Derivative1 ==
  f(t) : Inport
  Add : Sum  Inputs=+-  OutScaling=2^-10
  Constant : Constant  Value=5*T  OutDataTypeMode=single
  Divide : Product  Inputs=*/  OutScaling=2^-10
  Integer Delay : simulink/Discrete/Integer Delay  vinit=0.0  samptime=T  NumDelays=5
  f_dot(t) : Outport
  wires:
  Add/1 -> Divide/1
  f(t)/1 -> Add/1, Integer Delay/1
  Integer Delay/1 -> Add/2
  Constant/1 -> Divide/2
  Divide/1 -> f_dot(t)/1

== system InnerOuter_Sim/Navigation/Leg Run Computation/Pey > |L2| (Marius')/psi_dot to Bank ==
  psi_dot_c : Inport
  U_m : Inport  Port=2
  Constant1 : Constant  Value=9.80665  OutDataTypeMode=single
  Divide : Product  Inputs=**/  OutScaling=2^-10
  Subsystem2 : Subsystem  AncestorBlock=SLUGS_Library/Subsystem2
  phi_c : Outport
  wires:
  Divide/1 -> Subsystem2/1(x)
  Subsystem2/1(atan(x)) -> phi_c/1
  Constant1/1 -> Divide/3
  U_m/1 -> Divide/2
  psi_dot_c/1 -> Divide/1

== system InnerOuter_Sim/Navigation/Mode Determination/Recent Enable/Grab Upon Enable ==
  Puav : Inport
  Enable : EnablePort
  UAVic : Outport
  wires:
  Puav/1 -> UAVic/1

== system InnerOuter_Sim/Navigation/Mode Determination/Recent Enable/Subsystem ==
  WP Fly : Inport
  Add1 : Sum  Inputs=2  OutScaling=2^-10
  Hit  Crossing1 : HitCross  HitCrossingOffset=0.5  HitCrossingDirection=rising  SampleTime=apSampleTime
  Integer Delay1 : simulink/Discrete/Integer Delay  vinit=0  samptime=-1  NumDelays=1
  Just Enab : Outport
  wires:
  WP Fly/1 -> Hit  Crossing1/1
  Add1/1 -> Just Enab/1
  Hit  Crossing1/1 -> Integer Delay1/1, Add1/2
  Integer Delay1/1 -> Add1/1

== system InnerOuter_Sim/Navigation/Waypoint Transition Computation/Compute P/Compute R ==
  U_com : Inport
  Product : Product  OutDataTypeMode=single  RndMeth=Zero
  Product1 : Product  Inputs=*/  OutDataTypeMode=single  RndMeth=Zero
  gravity1 : Constant  Value=ISA_g*tan(bankCommandLimit)  OutDataTypeMode=single
  R : Outport
  wires:
  Product/1 -> Product1/1
  gravity1/1 -> Product1/2
  U_com/1 -> Product/1, Product/2
  Product1/1 -> R/1

== system InnerOuter_Sim/Navigation/Waypoint Transition Computation/Compute P/Get Circles ==
  T1 : Inport
  T2 : Inport  Port=2
  "Wp_to " : Inport  Port=3
  R : Inport  Port=4
  Compute  Circles : Stateflow chart
  Compute CCW Angle From 2 Vectors : Subsystem
  Compute delta Left Turn : Subsystem
  Constant5 : Constant  Value=pi  OutDataTypeMode=single
  Larger than 180? : RelationalOperator  LogicOutDataTypeMode=Boolean  LogicDataType=double()
  Logical Operator : Logic  Operator=NOT  AllPortsSameDT=off  OutDataTypeMode=Boolean
  Merge4 : Merge
  Subsystem5 : SLUGS_Library/Subsystem5  SystemSampleTime=-1
  To Workspace : ToWorkspace  VariableName=O  SampleTime=-1  SaveFormat=Structure
  To Workspace1 : ToWorkspace  VariableName=P  SampleTime=-1  SaveFormat=Structure
  To Workspace2 : ToWorkspace  VariableName=Pch  SampleTime=-1  SaveFormat=Structure
  To Workspace3 : ToWorkspace  VariableName=PchB  SampleTime=-1  SaveFormat=Structure
  compute delta Right Turn : Subsystem
  P : Outport
  wires:
  Subsystem5/2 -> Compute  Circles/2(cd)
  Subsystem5/1 -> Compute  Circles/1(sd)
  Logical Operator/1 -> Compute delta Left Turn/Enable
  Larger than 180?/1 -> Logical Operator/1, compute delta Right Turn/Enable
  Constant5/1 -> Larger than 180?/2
  Compute  Circles/4(PchB) -> To Workspace3/1
  Compute  Circles/3(Pch) -> To Workspace2/1
  Compute  Circles/2(P) -> To Workspace1/1, P/1
  Compute  Circles/1(O) -> To Workspace/1
  "Wp_to "/1 -> Compute  Circles/3(WP1)
  R/1 -> Compute  Circles/4(R)
  Compute delta Left Turn/1(delta) -> Merge4/2
  compute delta Right Turn/1(delta) -> Merge4/1
  Merge4/1 -> Subsystem5/1
  T2/1 -> Compute CCW Angle From 2 Vectors/2(V), Compute  Circles/6(T2)
  Compute CCW Angle From 2 Vectors/1(CCW Ang) -> Larger than 180?/1, compute delta Right Turn/1(gamma), Compute delta Left Turn/1(gamma)  "gamma"
  T1/1 -> Compute CCW Angle From 2 Vectors/1(U), Compute  Circles/5(T1)

== system InnerOuter_Sim/Navigation/Waypoint Transition Computation/Compute Total Run/Compute Distance ==
  Pos 1 : Inport
  Pos 2 : Inport  Port=2
  Add : Sum  Inputs=+-  OutScaling=2^-10
  Norm : Subsystem  AncestorBlock=SLUGS_Library/Navigation/Norm
  Dist : Outport
  wires:
  Pos 1/1 -> Add/1
  Pos 2/1 -> Add/2
  Add/1 -> Norm/1(Vector)
  Norm/1(Norm) -> Dist/1

== system InnerOuter_Sim/Navigation/Waypoint Transition Computation/Compute Total Run/Protect NaNs ==
  In1 : Inport
  Integer Delay3 : simulink/Discrete/Integer Delay  Orientation=left  vinit=0.0  samptime=T  NumDelays=1
  Relational Operator2 : RelationalOperator  Operator===  LogicOutDataTypeMode=Specify via dialog
  Switch3 : Switch  Criteria=u2 > Threshold  Threshold=0.3  SampleTime=.01
  Out1 : Outport  Orientation=down
  wires:
  Integer Delay3/1 -> Switch3/3
  Switch3/1 -> Out1/1, Integer Delay3/1
  In1/1 -> Relational Operator2/2, Relational Operator2/1, Switch3/1
  Relational Operator2/1 -> Switch3/2

== system InnerOuter_Sim/Navigation/Waypoint Transition Computation/Get Wps Compute Frenet1/Compute Frenet ==
  Pos 1 : Inport
  Pos 2 : Inport  Port=2
  Add : Sum  Inputs=-+  OutScaling=2^-10
  Normalize Vector : SLUGS_Library/Navigation/Normalize Vector  SystemSampleTime=-1
  "Normalize Vector " : SLUGS_Library/Navigation/Normalize Vector  SystemSampleTime=-1
  Select N  Terms : Stateflow chart
  Select N  Terms1 : Stateflow chart
  T : Outport
  N : Outport  Port=2
  wires:
  Pos 1/1 -> Add/1
  Pos 2/1 -> Add/2
  Add/1 -> Select N  Terms1/1(Tin)
  Select N  Terms/1(N) -> "Normalize Vector "/1
  "Normalize Vector "/1 -> N/1
  Normalize Vector/1 -> T/1, Select N  Terms/1(T)
  Select N  Terms1/1(T) -> Normalize Vector/1

== system InnerOuter_Sim/Navigation/Waypoint Transition Computation/Get Wps Compute Frenet1/Compute Frenet  ==
  Pos 1 : Inport
  Pos 2 : Inport  Port=2
  Add : Sum  Inputs=-+  OutScaling=2^-10
  Normalize Vector : SLUGS_Library/Navigation/Normalize Vector  SystemSampleTime=-1
  "Normalize Vector " : SLUGS_Library/Navigation/Normalize Vector  SystemSampleTime=-1
  Select N  Terms : Stateflow chart
  Select N  Terms1 : Stateflow chart
  T : Outport
  N : Outport  Port=2
  wires:
  Select N  Terms1/1(T) -> Normalize Vector/1
  Normalize Vector/1 -> Select N  Terms/1(T), T/1
  "Normalize Vector "/1 -> N/1
  Select N  Terms/1(N) -> "Normalize Vector "/1
  Add/1 -> Select N  Terms1/1(Tin)
  Pos 2/1 -> Add/2
  Pos 1/1 -> Add/1

== system InnerOuter_Sim/Navigation/Waypoint Transition Computation/Get Wps Compute Frenet1/get WP Coord from Index ==
  WP Idx : Inport
  C Function Call : dsPICdrivers/OTHERS/C Function Call  Tag=dsPIC_dsPIC_CFunctionCall  fctName='getWP'  INPUT_SIZE=1  INPUT1=uint8  INPUT2=--  INPUT3=--  OUTPUT_SIZE=3  OUTPUT1=real32  SampleTime=-1  InputType=[ 2 ]  OutputType=[ 7 ]  FctDeclaration=extern void getWP(uint8_T u1,real32_T* y1);  FctCall=getWP(%u1, *%y1);  OrderingInOutPopup=None
  Data Type Conversion : DataTypeConversion  OutDataTypeMode=double
  Data Type Conversion1 : DataTypeConversion  OutDataTypeMode=single
  Environment Controller : simulink/Signal Routing/Environment Controller  SystemSampleTime=-1
  MATLAB Fcn : MATLABFcn  MATLABFcn=Xpoints(u(1))  OutputDimensions=1  OutputSignalType=real
  MATLAB Fcn1 : MATLABFcn  MATLABFcn=Ypoints(u(1))  OutputDimensions=1
  MATLAB Fcn2 : MATLABFcn  MATLABFcn=Zpoints(u(1))  OutputDimensions=1
  Mux : Mux  Inputs=3
  WP Coord : Outport
  wires:
  Data Type Conversion1/1 -> Environment Controller/1
  Data Type Conversion/1 -> MATLAB Fcn2/1, MATLAB Fcn/1, MATLAB Fcn1/1
  MATLAB Fcn/1 -> Mux/1
  MATLAB Fcn1/1 -> Mux/2
  MATLAB Fcn2/1 -> Mux/3
  WP Idx/1 -> Data Type Conversion/1, C Function Call/1
  Mux/1 -> Data Type Conversion1/1
  Environment Controller/1 -> WP Coord/1
  C Function Call/1 -> Environment Controller/2

== system InnerOuter_Sim/Navigation/Waypoint Transition Computation/Get Wps Compute Frenet1/get WP Coord from Index  ==
  WP Idx : Inport
  C Function Call : dsPICdrivers/OTHERS/C Function Call  Tag=dsPIC_dsPIC_CFunctionCall  fctName='getWP'  INPUT_SIZE=1  INPUT1=uint8  INPUT2=--  INPUT3=--  OUTPUT_SIZE=3  OUTPUT1=real32  SampleTime=-1  InputType=[ 2 ]  OutputType=[ 7 ]  FctDeclaration=extern void getWP(uint8_T u1,real32_T* y1);  FctCall=getWP(%u1, *%y1);  OrderingInOutPopup=None
  Data Type Conversion : DataTypeConversion  OutDataTypeMode=double
  Data Type Conversion1 : DataTypeConversion  OutDataTypeMode=single
  Environment Controller : simulink/Signal Routing/Environment Controller  SystemSampleTime=-1
  MATLAB Fcn : MATLABFcn  MATLABFcn=Xpoints(u(1))  OutputDimensions=1  OutputSignalType=real
  MATLAB Fcn1 : MATLABFcn  MATLABFcn=Ypoints(u(1))  OutputDimensions=1
  MATLAB Fcn2 : MATLABFcn  MATLABFcn=Zpoints(u(1))  OutputDimensions=1
  Mux : Mux  Inputs=3
  WP Coord : Outport
  wires:
  Data Type Conversion1/1 -> Environment Controller/1
  Data Type Conversion/1 -> MATLAB Fcn2/1, MATLAB Fcn/1, MATLAB Fcn1/1
  MATLAB Fcn/1 -> Mux/1
  MATLAB Fcn1/1 -> Mux/2
  MATLAB Fcn2/1 -> Mux/3
  WP Idx/1 -> Data Type Conversion/1, C Function Call/1
  Mux/1 -> Data Type Conversion1/1
  Environment Controller/1 -> WP Coord/1
  C Function Call/1 -> Environment Controller/2

== system InnerOuter_Sim/Navigation/Waypoint Transition Computation/Get Wps Compute Frenet1/get WP Coord from Index    ==
  WP Idx : Inport
  C Function Call : dsPICdrivers/OTHERS/C Function Call  Tag=dsPIC_dsPIC_CFunctionCall  fctName='getWP'  INPUT_SIZE=1  INPUT1=uint8  INPUT2=--  INPUT3=--  OUTPUT_SIZE=3  OUTPUT1=real32  SampleTime=-1  InputType=[ 2 ]  OutputType=[ 7 ]  FctDeclaration=extern void getWP(uint8_T u1,real32_T* y1);  FctCall=getWP(%u1, *%y1);  OrderingInOutPopup=None
  Data Type Conversion : DataTypeConversion  OutDataTypeMode=double
  Data Type Conversion1 : DataTypeConversion  OutDataTypeMode=single
  Environment Controller : simulink/Signal Routing/Environment Controller  SystemSampleTime=-1
  MATLAB Fcn : MATLABFcn  MATLABFcn=Xpoints(u(1))  OutputDimensions=1  OutputSignalType=real
  MATLAB Fcn1 : MATLABFcn  MATLABFcn=Ypoints(u(1))  OutputDimensions=1
  MATLAB Fcn2 : MATLABFcn  MATLABFcn=Zpoints(u(1))  OutputDimensions=1
  Mux : Mux  Inputs=3
  WP Coord : Outport
  wires:
  C Function Call/1 -> Environment Controller/2
  Environment Controller/1 -> WP Coord/1
  Mux/1 -> Data Type Conversion1/1
  WP Idx/1 -> C Function Call/1, Data Type Conversion/1
  MATLAB Fcn2/1 -> Mux/3
  MATLAB Fcn1/1 -> Mux/2
  MATLAB Fcn/1 -> Mux/1
  Data Type Conversion/1 -> MATLAB Fcn1/1, MATLAB Fcn/1, MATLAB Fcn2/1
  Data Type Conversion1/1 -> Environment Controller/1

== system InnerOuter_Sim/6DOF Model/Plant/6-DOF EOM/[V1,2,3,W1,2,3]/A = [M ; J] ==
  Constant1 : Constant  Value=zeros(3,3)
  Constant4 : Constant  Value=0
  Display : Display
  Display1 : Display
  Display2 : Display
  Ixx : Constant  Value=Ixx  VectorParams1D=off
  Iyy : Constant  Value=Iyy  VectorParams1D=off
  Izz : Constant  Value=Izz  VectorParams1D=off
  Matrix Concatenation : Concatenate  Mode=Multidimensional array
  Matrix Concatenation1 : Concatenate  Mode=Multidimensional array
  Matrix Concatenation2 : Concatenate  Mode=Multidimensional array  ConcatenateDimension=2
  Mux : Mux  Inputs=9
  Mux1 : Mux  Inputs=9
  Reshape : Reshape  OutputDimensionality=Customize  OutputDimensions=[3,3]
  Reshape1 : Reshape  OutputDimensionality=Customize  OutputDimensions=[3,3]
  mass : Constant  Value=mass  VectorParams1D=off
  A Matrix : Outport
  wires:
  Ixx/1 -> Mux/1
  Izz/1 -> Mux/9
  Iyy/1 -> Mux/5
  Constant4/1 -> Mux/8, Mux/7, Mux/6, Mux/4, Mux/3, Mux/2, Mux1/8, Mux1/7, Mux1/6, Mux1/4, Mux1/3, Mux1/2
  mass/1 -> Mux1/1, Mux1/5, Mux1/9
  Mux1/1 -> Reshape/1
  Mux/1 -> Reshape1/1
  Matrix Concatenation/1 -> Matrix Concatenation2/1, Display/1
  Matrix Concatenation1/1 -> Matrix Concatenation2/2, Display1/1
  Matrix Concatenation2/1 -> A Matrix/1, Display2/1
  Reshape1/1 -> Matrix Concatenation1/2
  Reshape/1 -> Matrix Concatenation/1
  Constant1/1 -> Matrix Concatenation/2, Matrix Concatenation1/1

== system InnerOuter_Sim/6DOF Model/Plant/6-DOF EOM/[V1,2,3,W1,2,3]/Get Grav Force in Body ==
  Euler : Inport
  Grav Force : Inport  Port=2
  Math Function : Math  Operator=transpose  SaturateOnIntegerOverflow=on
  Product1 : Product  Multiplication=Matrix(*)  SaturateOnIntegerOverflow=on  InputSameDT=on
  Rb2u : Subsystem
  Reshape : Reshape  OutputDimensionality=Column vector (2-D)
  Grav Force (Body) : Outport
  wires:
  Rb2u/1(DCM) -> Math Function/1
  Euler/1 -> Rb2u/1(phi theta psi)
  Product1/1 -> Grav Force (Body)/1
  Math Function/1 -> Product1/1
  Grav Force/1 -> Reshape/1
  Reshape/1 -> Product1/2

== system InnerOuter_Sim/6DOF Model/Plant/6-DOF EOM/[V1,2,3,W1,2,3]/Sigma ==
  note: S(pqr)
  pqr : Inport
  Gain : Gain  Gain=[0 0 0;0 0 -1; 0 1 0]  Multiplication=Matrix(K*u)  SaturateOnIntegerOverflow=on
  Gain1 : Gain  Gain=[0 0 1;0 0 0; -1 0 0]  Multiplication=Matrix(K*u)  SaturateOnIntegerOverflow=on
  Gain2 : Gain  Gain="[0 -1 0;1 0 0;  0 0 0]"  Multiplication=Matrix(K*u)  SaturateOnIntegerOverflow=on
  Gain3 : Gain  Gain=0  SaturateOnIntegerOverflow=on
  Math Function : Math  Operator=transpose  SaturateOnIntegerOverflow=on
  Matrix Concatenation : Concatenate  Mode=Multidimensional array  ConcatenateDimension=2
  Matrix Concatenation1 : Concatenate  Mode=Multidimensional array  ConcatenateDimension=2
  Matrix Concatenation2 : Concatenate  Mode=Multidimensional array
  Mux : Mux  Inputs=3
  Reshape : Reshape  OutputDimensionality=Customize  OutputDimensions=[3,3]
  Sigma : Outport
  wires:
  Mux/1 -> Reshape/1
  Gain/1 -> Mux/1
  Gain1/1 -> Mux/2
  Gain2/1 -> Mux/3
  Reshape/1 -> Math Function/1
  Math Function/1 -> Gain3/1, Matrix Concatenation/1, Matrix Concatenation1/2
  Gain3/1 -> Matrix Concatenation/2, Matrix Concatenation1/1
  Matrix Concatenation/1 -> Matrix Concatenation2/1
  Matrix Concatenation1/1 -> Matrix Concatenation2/2
  Matrix Concatenation2/1 -> Sigma/1
  pqr/1 -> Gain/1, Gain2/1, Gain1/1

== system InnerOuter_Sim/6DOF Model/Plant/Forces and Moments/Body Frame F & M/Transfer to body frame ==
  Wind frame  F&M : Inport
  "aoa/beta, deg" : Inport  Port=2
  D2R : Gain  Gain=pi/180  SaturateOnIntegerOverflow=on
  Forces : Selector  IndexOptions=Index vector (dialog)  Indices=[1 2 3]  OutputSizes=[(-2)]  InputPortWidth=6
  Moments : Selector  IndexOptions=Index vector (dialog)  Indices=[4 5 6]  OutputSizes=[(-2)]  InputPortWidth=6
  Ra2b1 : Subsystem
  Ra2b22 : Subsystem
  Scope : Scope
      settings: YMin=-450  YMax=200  SaveName=ScopeData11
  Scope1 : Scope
      settings: YMin=-450  YMax=200  SaveName=ScopeData17
  F_b : Outport
  M_b : Outport  Port=2
  wires:
  Ra2b1/1(body frame) -> F_b/1, Scope/1  "Fb"
  Ra2b22/1(body frame) -> Scope1/1, M_b/1  "Mb"
  "aoa/beta, deg"/1 -> D2R/1
  Forces/1 -> Ra2b1/1(wind frame)
  Wind frame  F&M/1 -> Forces/1, Moments/1
  Moments/1 -> Ra2b22/2(wind frame)
  D2R/1 -> Ra2b1/2(aoa/beta), Ra2b22/1(aoa/beta)
